simulink model "Modello_Simulink_Dirigibile"  (R2013a)
settings: Solver=ode45  StartTime=0.0  StopTime=10.0  RelTol=1e-3
libraries: dspsigops x1
settings Model: Creator=training-it  LastModifiedBy=Pera
settings DataIOCC: SignalLoggingSaveFormat=ModelDataLogs
settings DebuggingCC: MultiTaskDSMMsg=warning  MultiTaskCondExecSysMsg=none  StateNameClashWarn=none  StrictBusMsg=None
settings RTWCC: IncludeERTFirstTime=on

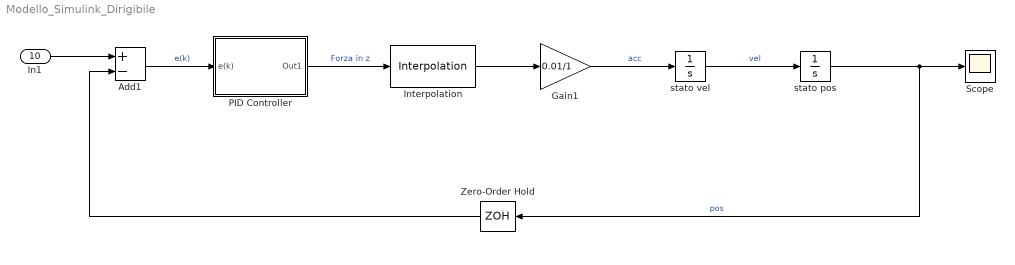
== system Modello_Simulink_Dirigibile ==
  In1 : Inport  Port=10
  Add1 : Sum  Inputs=+-
  Gain1 : Gain  Gain=0.01/1
  Interpolation : dspsigops/Interpolation  InterpSource=Specify via dialog  InterpPoints=[1.1 4.8 2.67 1.6 3.2]'  InterpMode=FIR  InterpL=3  InterpR=3  InterpAlpha=0.5  InvalidMode=Clip
  PID Controller : Subsystem  mask{Ts=0.1, kp=0.3, ki=2, kd=0.1}
      mask prompts: Ts "Sample Time"; kp "Guadagno Proporzionale"; ki "Guadagno Integrativo"; kd "Guadagno Derivativo"
      mask init:
      | s1=['kp= ',num2str(kp)];
      | s2=['ki= ',num2str(ki)];
      | s3=['kd= ',num2str(ki)];
      | s=strvcat(s1,s2,s3);  %sto concatenando verticalmente
      mask Display: disp(s)
  Scope : Scope
  Zero-Order Hold : ZeroOrderHold  SampleTime=0.1
  stato pos : Integrator  InitialCondition=x0  mask{x0=0}
      mask prompts: x0 "posizione iniziale"
  stato vel : Integrator  mask{v0=0}
      mask prompts: v0 "velocità iniziale"
  wires:
  stato vel/1 -> stato pos/1  "vel"
  stato pos/1 -> Scope/1, Zero-Order Hold/1  "pos"
  In1/1 -> Add1/1
  Add1/1 -> PID Controller/1(e(k))  "e(k)"
  PID Controller/1(Out1) -> Interpolation/1  "Forza in z"
  Gain1/1 -> stato vel/1  "acc"
  Zero-Order Hold/1 -> Add1/2
  Interpolation/1 -> Gain1/1

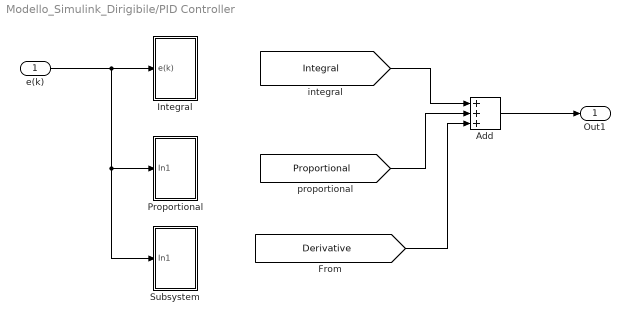
== system Modello_Simulink_Dirigibile/PID Controller ==
  e(k) : Inport
  Add : Sum  Inputs=+++
  Integral : Subsystem
  Proportional : Subsystem
  Subsystem : Subsystem
  Out1 : Outport
  wires:
  [Integral] -> Add/1
  Add/1 -> Out1/1
  [Proportional] -> Add/2
  e(k)/1 -> Subsystem/1(In1), Proportional/1(In1), Integral/1(e(k))
  [Derivative] -> Add/3

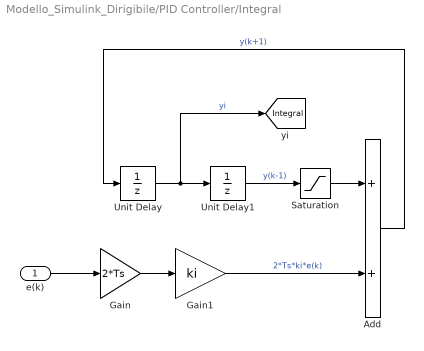
== system Modello_Simulink_Dirigibile/PID Controller/Integral ==
  e(k) : Inport
  Add : Sum
  Gain : Gain  Gain=2*Ts
  Gain1 : Gain  Gain=ki
  Saturation : Saturate  UpperLimit=1  LowerLimit=-1
      settings: AttributesFormatString=|
      | %<LowerLimit>
      | %<UpperLimit>
  Unit Delay : UnitDelay  SampleTime=Ts
  Unit Delay1 : UnitDelay  SampleTime=Ts
  tag scope: Integral=global
  wires:
  Gain1/1 -> Add/2  "2*Ts*ki*e(k)"
  Unit Delay/1 -> [Integral], Unit Delay1/1  "yi"
  Gain/1 -> Gain1/1
  Saturation/1 -> Add/1
  Unit Delay1/1 -> Saturation/1  "y(k-1)"
  e(k)/1 -> Gain/1
  Add/1 -> Unit Delay/1  "y(k+1)"

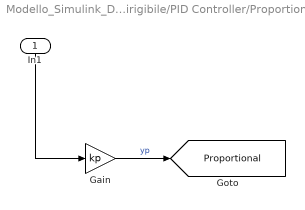
== system Modello_Simulink_Dirigibile/PID Controller/Proportional ==
  In1 : Inport
  Gain : Gain  Gain=kp
  tag scope: Proportional=global
  wires:
  Gain/1 -> [Proportional]  "yp"
  In1/1 -> Gain/1

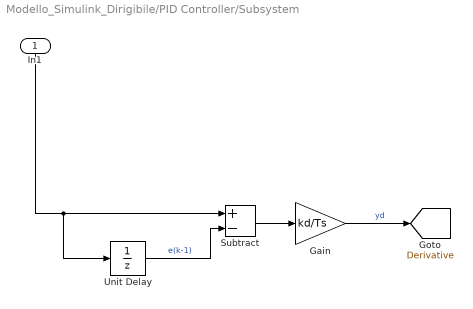
== system Modello_Simulink_Dirigibile/PID Controller/Subsystem ==
  In1 : Inport
  Gain : Gain  Gain=kd/Ts
  Subtract : Sum  Inputs=+-
  Unit Delay : UnitDelay  SampleTime=-1
  tag scope: Derivative=global
  wires:
  Unit Delay/1 -> Subtract/2  "e(k-1)"
  Gain/1 -> [Derivative]  "yd"
  Subtract/1 -> Gain/1
  In1/1 -> Unit Delay/1, Subtract/1
